simulink model "nms_3Dmodel_mld"  (R2019a)
settings: Solver=ode15s  StartTime=0.0  StopTime=7  FixedStep=1e-3  RelTol=1e-3  AbsTol=1e-4  EnableMultiTasking=on
InitFcn:
  | runScripts;
undefined symbols (not defined in the file or in its folder): ankle_height, c, c_jointstop, CtrlPar_FP, CtrlPar_FP_R, CtrlPar_LL, CtrlPar_St, CtrlPar_St_R, CtrlPar_Sw, CtrlPar_Sw_R, CtrlPar_theta0, CtrlPar_Tr, CtrlPar_Tr_R, D12_F, D12_S, D12_T, D12z_T, D13_F, D1G_F, D1G_HAT, D1G_S, D1G_T, D1Gy_F, d_fBall, d_fHeel, DeltaThRef, dt, eref, FmaxBFSH, FmaxGAS, FmaxGLU, FmaxHAB, FmaxHAD, FmaxHAM, FmaxHFL, FmaxRF, FmaxSOL, FmaxTA, FmaxVAS, In_F, In_HAT, In_S, In_T, init_a_tgt, init_a_tgtR, Inx_F, Inx_HAT, Inx_S, Inx_T, Iny_F, Iny_HAT, Iny_S, Iny_T, K, k_gn, k_gt, k_pressure, leg_l, LongDelay, LongLoopDelay ... (+139)
libraries: mblibv1 x89, simulink x44, simulink_extras x38
(part 2 of 13)

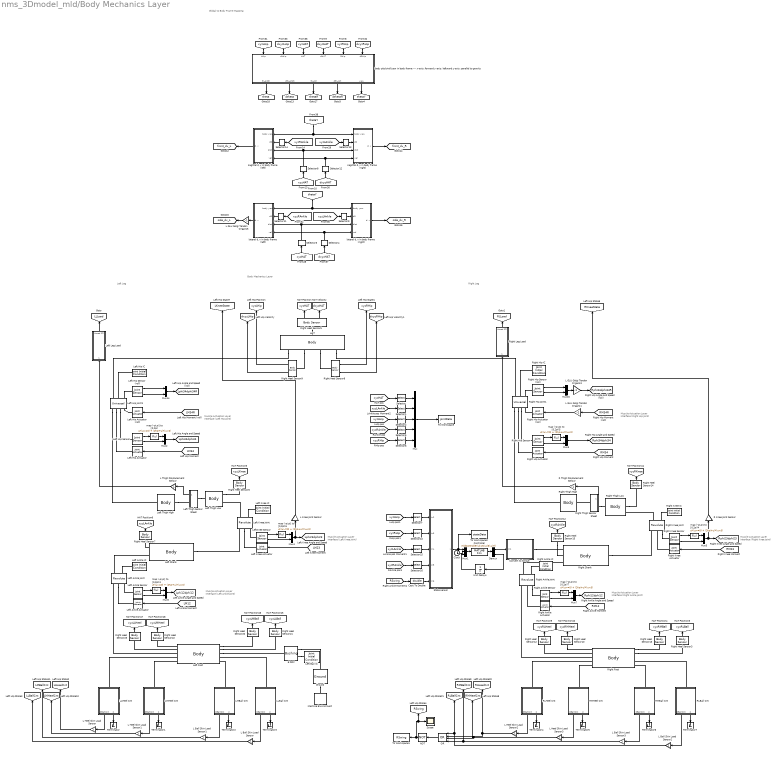
== system nms_3Dmodel_mld/Body Mechanics Layer ==
  note: Body Mechanics Layer
  note: Left Leg
  note: Right Leg
  note: Muscle Actuation
      | Layer Interface
      | (Left Hip Joint)
  note: Muscle Actuation
      | Layer Interface
      | (Left Knee Joint)
  note: Muscle Actuation
      | Layer Interface
      | (Left Ankle Joint)
  note: Muscle Actuation
      | Layer Interface
      | (Right Ankle Joint)
  note: Muscle Actuation
      | Layer Interface
      | (Right Knee Joint)
  note: Muscle Actuation
      | Layer Interface
      | (Right Hip Joint)
  note: Global to Body Frame Mapping
  6 DOF : mblibv1/Joints/Bushing  LConnTagsString=__newl0|SA1  RConnTagsString=__newr0  UpdateFromCAD=off  NumSAPorts=1  CutJoint=off  MarkAsCut=off  Primitives=prismatic_prismatic_prismatic  PrimitiveProps=P1$World$[1 0 0]$prismatic#P2$World$[0 1 0]$prismatic#P3$World$[0 0 1]$prismatic#R1$World$[1 0 0]$revolute#R2$World$[0 1 0]$revolute#R3$World$[0 0 1]$revolute  DialogClass=JointBlock  P1Axis=[1 0 0]  P2Axis=[0 1 0]  P3Axis=[0 0 1]  R1Axis=[1 0 0]  R2Axis=[0 1 0]  R3Axis=[0 0 1]
      settings: SourceProductName=Simscape Multibody  SourceProductBaseCode=MS
  Cast To Double : DataTypeConversion  OutDataTypeStr=double
  Clock : Clock
  Controller : MATLABFcn  MATLABFcn=mldController(u(1:5),u(6),u(7))  OutputDimensions=2  SampleTime=0.01
  "Convert to torque " : Subsystem
  Demux : Demux  Outputs=2
  Ground : mblibv1/Bodies/Ground  UpdateFromCAD=off  LeftPortType=env  RightPortType=workingframe  PhysicalDomain=Mechanical  DialogClass=GroundBlock  CoordPosition=[0 0 0]  CoordPositionUnits=m  StateVectorMgrId=1  MachineId=[2 0]  ShowEnvPort=on  ParameterChecksum=[2753857904, 2875425358, 3568229323, 1209649953]  TopologyChecksum=[3539625464, 3223322067, 2116753285, 3317004890]
      settings: SourceProductName=Simscape Multibody  SourceProductBaseCode=MS
  HAT : mblibv1/Bodies/Body  LConnTagsString=CG  RConnTagsString=CS1|CS2|CS3|CS4  UpdateFromCAD=off  DialogClass=MechanicalBodyBlock  Mass=m_HAT  MassUnits=kg  InertiaUnits=kg*m^2  Inertia=[Inx_HAT 0 0; 0 Iny_HAT 0; 0 0 In_HAT]  Shape=Cylinder  ShapeDims=[1 1]  ShapeUnits=m  ShapeUse=false  Density=1  DensityUnits=kg/m^3  DensityUse=false  GraphicsMode=MACHINE_DEFAULT  BodyColorSelMode=MACHINE_DEFAULT  BodyColor=[1 0 0]  AttachedToCS=CG  CG=Left$CG$[D1G_HAT 0 D12z_T]$CS1$CS1$m$[0 0 0]$Euler X-Y-Z$deg$WORLD$true$none  WorkingFrames=Left$CS5$[0.8 0 D12z_T]$CS1$CS1$m$[0 0 0]$Euler X-Y-Z$deg$WORLD$false$none#Right$CS1$[0 0 0]$ADJOINING$ADJOINING$m$[0 0 0]$Euler X-Y-Z$deg$WORLD$true$none#Right$CS2$[0 0 0]$CS1$CS1$m$[0 0 0]$Euler X-Y-Z$deg$WORLD$true$none#Right$CS3$[0 0 0]$CS4$CS4$m$[0 0 0]$Euler X-Y-Z$deg$WORLD$true$none#Right$CS4$[0 0 2*D12z_T]$CS1$CS1$m$[0 0 0]$Euler X-Y-Z$deg$WORLD$true$none  CGPos=[D1G_HAT 0 D12z_T]  CGRot=[0 0 0]  CS0Pos=[]  CS0Rot=[]  CS1Pos=[0 0 0]  CS1Rot=[0 0 0]  CS2Pos=[0 0 0]  CS2Rot=[0 0 0]  CS3Pos=[0 0 0]  CS3Rot=[0 0 0]  CS4Pos=[0 0 2*D12z_T]  CS4Rot=[0 0 0]  CS5Pos=[0.8 0 D12z_T]  CS5Rot=[0 0 0]  CS6Pos=[]  CS6Rot=[]  CS7Pos=[]  CS7Rot=[]  CS8Pos=[]  CS8Rot=[]  CS9Pos=[]  CS9Rot=[]  CS10Pos=[]  CS10Rot=[]  CS11Pos=[]  CS11Rot=[]  CS12Pos=[]  CS12Rot=[]  CS13Pos=[]  CS13Rot=[]  CS14Pos=[]  CS14Rot=[]  CS15Pos=[]  CS15Rot=[]  CS16Pos=[]  CS16Rot=[]  CS17Pos=[]  CS17Rot=[]  CS18Pos=[]  CS18Rot=[]  CS19Pos=[]  CS19Rot=[]  CS20Pos=[]  CS20Rot=[]
      settings: SourceProductName=Simscape Multibody  SourceProductBaseCode=MS
  L Ball Skin Load Sensor{,1..3} (4 alike) : Gain
  L GLU Golgi Tendon Organs1 : Gain  Gain=-1
  L GLU Golgi Tendon Organs3 : Gain  Gain=-1
  L GLU Golgi Tendon Organs5 : Gain  Gain=-1
  L Heel Skin Load Sensor{,1..3} (4 alike) : Gain
  L Knee Joint Sensor : Gain
  L Thigh Displacement  Sensor : Gain
  LLBall Cnt : Subsystem
  LLHeel Cnt : Subsystem
  LMBall Cnt : Subsystem
  LMHeel Cnt : Subsystem
  Left Ankle Joint : mblibv1/Joints/Revolute  LConnTagsString=__newl0|SA1|SA2  RConnTagsString=__newr0|SA1  UpdateFromCAD=off  NumSAPorts=3  CutJoint=off  MarkAsCut=off  Primitives=revolute  PrimitiveProps=R1$WORLD$[0 0 1]$revolute  DialogClass=JointBlock  R1Axis=[0 0 1]
      settings: SourceProductName=Simscape Multibody  SourceProductBaseCode=MS
  Left Hip Joint1 : mblibv1/Joints/Universal  LConnTagsString=__newl0|SA1|SA2|SA3  RConnTagsString=__newr0|SA1|SA2  UpdateFromCAD=off  NumSAPorts=5  CutJoint=off  MarkAsCut=off  Primitives=prismatic  PrimitiveProps=R1$World$[0 0 1]$revolute#R2$World$[0 1 0]$revolute  DialogClass=JointBlock  R1Axis=[0 0 1]  R2Axis=[0 1 0]
      settings: SourceProductName=Simscape Multibody  SourceProductBaseCode=MS
  Left Knee Joint : mblibv1/Joints/Revolute  LConnTagsString=__newl0|SA1|SA2  RConnTagsString=__newr0|SA1  UpdateFromCAD=off  NumSAPorts=3  CutJoint=off  MarkAsCut=off  Primitives=revolute  PrimitiveProps=R1$WORLD$[0 0 -1]$revolute  DialogClass=JointBlock  R1Axis=[0 0 -1]
      settings: SourceProductName=Simscape Multibody  SourceProductBaseCode=MS
  Left Ankle Actuator : mblibv1/Sensors &  Actuators/Joint Actuator  UpdateFromCAD=off  PhysicalDomain=Mechanical  PortType=blob  ActuationStyle=Force  AngleUnits=deg  ArcVelocityUnits=deg/s  ArcAccelerationUnits=deg/s^2  CoordPositionUnits=m  VelocityUnits=m/s  AccelerationUnits=m/s^2  ForceUnits=N  TorqueUnits=N-m  ActiveIO=on  Width=1  DialogClass=MechanicalActuatorBlock  Primitive=R1  ReferenceFrame=Absolute (INERTIAL)
      settings: SourceProductName=Simscape Multibody  SourceProductBaseCode=MS
  Left Ankle Sensor : mblibv1/Sensors &  Actuators/Joint Sensor  UpdateFromCAD=off  PhysicalDomain=Mechanical  PortType=blob  Muxed=off  Pose=off  Angle=on  AngleUnits=rad  ArcVelocity=on  ArcVelocityUnits=rad/s  ArcAcceleration=off  ArcAccelerationUnits=deg/s^2  CoordPosition=on  CoordPositionUnits=m  Velocity=off  VelocityUnits=m/s  Acceleration=off  AccelerationUnits=m/s^2  Quaternion=on  QuaternionDT=off  QuaternionDDT=off  QuaternionUnits=off  OutputVector=[ 1 1 ]  ActiveIO=on  Width=2  DialogClass=MechanicalSensorBlock  Primitive=R1  Force=off  ForceUnits=N  Torque=off  TorqueUnits=N-m  ReferenceFrame=Absolute (INERTIAL)  ReactionSensedSide=Base  ReactionReferenceFrame=Absolute (World)  ReactionForce=off  ReactionForceUnits=N  ReactionMoment=off  ReactionMomentUnits=N-m
      settings: SourceProductName=Simscape Multibody  SourceProductBaseCode=MS
  Left Ankle IC : mblibv1/Sensors &  Actuators/Joint Initial Condition  UpdateFromCAD=off  LeftPortType=blob  RightPortType=blob  PhysicalDomain=mechanical  DialogClass=InitialConditionBlock  InitialConditions=P1$false$0$m$rad$0$m/s$rad/s#P2$false$0$m$rad$0$m/s$rad/s#P3$false$0$m$rad$0$m/s$rad/s#R1$true$Lphi120$m$rad$0$m/s$rad/s#R2$false$0$m$rad$0$m/s$rad/s#R3$false$0$m$rad$0$m/s$rad/s#S$false$0$m$rad$0$m/s$rad/s  P1PIC=0  P1VIC=0  P2PIC=0  P2VIC=0  P3PIC=0  P3VIC=0  R1PIC=Lphi120  R1VIC=0  R2PIC=0  R2VIC=0  R3PIC=0  R3VIC=0  SPIC=0  SVIC=0
      settings: SourceProductName=Simscape Multibody  SourceProductBaseCode=MS
  Left Ball IC : mblibv1/Sensors &  Actuators/Joint Initial Condition  UpdateFromCAD=off  LeftPortType=blob  RightPortType=blob  PhysicalDomain=mechanical  DialogClass=InitialConditionBlock  InitialConditions=P1$true$x0$m$deg$vx0$m/s$deg/s#P2$true$z0$m$deg$0$m/s$deg/s#P3$true$-y0$m$deg$-vy0$m/s$deg/s#R1$true$roll0$m$rad$0$m/s$rad/s#R2$true$yaw0$m$rad$0$m/s$rad/s#R3$false$0$m$rad$0$m/s$rad/s#S$false$0$m$deg$0$m/s$deg/s  P1PIC=x0  P1VIC=vx0  P2PIC=z0  P2VIC=0  P3PIC=-y0  P3VIC=-vy0  R1PIC=roll0  R1VIC=0  R2PIC=yaw0  R2VIC=0  R3PIC=0  R3VIC=0  SPIC=0  SVIC=0
      settings: SourceProductName=Simscape Multibody  SourceProductBaseCode=MS
  Left Foot : mblibv1/Bodies/Body  LConnTagsString=CS3|CS4|CS1|CS5|CS6  RConnTagsString=CS7|CS8|CS2|CS9|CS10  UpdateFromCAD=off  DialogClass=MechanicalBodyBlock  Mass=m_F  MassUnits=kg  InertiaUnits=kg*m^2  Inertia=[Inx_F 0 0; 0 Iny_F 0; 0 0 In_F]  Shape=Cylinder  ShapeDims=[1 1]  ShapeUnits=m  ShapeUse=false  Density=1  DensityUnits=kg/m^3  DensityUse=false  GraphicsMode=MACHINE_DEFAULT  BodyColorSelMode=MACHINE_DEFAULT  BodyColor=[1 0 0]  AttachedToCS=CG  CG=Left$CG$[-D1G_F D1Gy_F 0]$CS1$CS1$m$[0 0 0]$Euler X-Y-Z$deg$WORLD$false$none  WorkingFrames=Left$CS3$[0 0 d_fBall/2]$CS1$CS1$m$[0 0 0]$Euler X-Y-Z$deg$WORLD$true$none#Left$CS4$[0 0 -d_fBall/2]$CS1$CS1$m$[0 0 0]$Euler X-Y-Z$deg$WORLD$true$none#Right$CS7$[-D13_F 0 d_fHeel/2]$CS1$CS1$m$[0 0 0]$Euler X-Y-Z$deg$WORLD$true$none#Right$CS8$[-D13_F 0 -d_fHeel/2]$CS1$CS1$m$[0 0 0]$Euler X-Y-Z$deg$WORLD$true$none#Left$CS1$[0 0 0]$ADJOINING$ADJOINING$m$[0 0 0]$Euler X-Y-Z$deg$WORLD$true$none#Right$CS2$[-D12_F ankle_height 0]$CS1$CS1$m$[0 0 0]$Euler X-Y-Z$deg$WORLD$true$none#Left$CS5$[0 0 0]$CS4$CS4$m$[0 0 0]$Euler X-Y-Z$deg$WORLD$true$none#Left$CS6$[0 0 0]$CS3$CS3$m$[0 0 0]$Euler X-Y-Z$deg$WORLD$true$none#Right$CS9$[0 0 0]$CS8$CS8$m$[0 0 0]$Euler X-Y-Z$deg$WORLD$true$none#Right$CS10$[0 0 0]$CS7$CS7$m$[0 0 0]$Euler X-Y-Z$deg$WORLD$true$none  CGPos=[-D1G_F D1Gy_F 0]  CGRot=[0 0 0]  CS0Pos=[]  CS0Rot=[]  CS1Pos=[0 0 0]  CS1Rot=[0 0 0]  CS2Pos=[-D12_F ankle_height 0]  CS2Rot=[0 0 0]  CS3Pos=[0 0 d_fBall/2]  CS3Rot=[0 0 0]  CS4Pos=[0 0 -d_fBall/2]  CS4Rot=[0 0 0]  CS5Pos=[0 0 0]  CS5Rot=[0 0 0]  CS6Pos=[0 0 0]  CS6Rot=[0 0 0]  CS7Pos=[-D13_F 0 d_fHeel/2]  CS7Rot=[0 0 0]  CS8Pos=[-D13_F 0 -d_fHeel/2]  CS8Rot=[0 0 0]  CS9Pos=[0 0 0]  CS9Rot=[0 0 0]  CS10Pos=[0 0 0]  CS10Rot=[0 0 0]  CS11Pos=[]  CS11Rot=[]  CS12Pos=[]  CS12Rot=[]  CS13Pos=[]  CS13Rot=[]  CS14Pos=[]  CS14Rot=[]  CS15Pos=[]  CS15Rot=[]  CS16Pos=[]  CS16Rot=[]  CS17Pos=[]  CS17Rot=[]  CS18Pos=[]  CS18Rot=[]  CS19Pos=[]  CS19Rot=[]  CS20Pos=[]  CS20Rot=[]
      settings: SourceProductName=Simscape Multibody  SourceProductBaseCode=MS
  Left Hip Actuator : mblibv1/Sensors &  Actuators/Joint Actuator  UpdateFromCAD=off  PhysicalDomain=Mechanical  PortType=blob  ActuationStyle=Force  AngleUnits=deg  ArcVelocityUnits=deg/s  ArcAccelerationUnits=deg/s^2  CoordPositionUnits=m  VelocityUnits=m/s  AccelerationUnits=m/s^2  ForceUnits=N  TorqueUnits=N-m  ActiveIO=on  Width=1  DialogClass=MechanicalActuatorBlock  Primitive=R1  ReferenceFrame=Absolute (INERTIAL)
      settings: SourceProductName=Simscape Multibody  SourceProductBaseCode=MS
  Left Hip Actuator (roll) : mblibv1/Sensors &  Actuators/Joint Actuator  UpdateFromCAD=off  PhysicalDomain=Mechanical  PortType=blob  ActuationStyle=Force  AngleUnits=rad  ArcVelocityUnits=rad/s  ArcAccelerationUnits=rad/s^2  CoordPositionUnits=m  VelocityUnits=m/s  AccelerationUnits=m/s^2  ForceUnits=N  TorqueUnits=N*m  ActiveIO=on  Width=1  DialogClass=MechanicalActuatorBlock  Primitive=R2  ReferenceFrame=Absolute (INERTIAL)
      settings: SourceProductName=Simscape Multibody  SourceProductBaseCode=MS
  Left Hip Sensor : mblibv1/Sensors &  Actuators/Joint Sensor  UpdateFromCAD=off  PhysicalDomain=Mechanical  PortType=blob  Muxed=off  Pose=off  Angle=on  AngleUnits=rad  ArcVelocity=on  ArcVelocityUnits=rad/s  ArcAcceleration=off  ArcAccelerationUnits=deg/s^2  CoordPosition=on  CoordPositionUnits=m  Velocity=on  VelocityUnits=m/s  Acceleration=off  AccelerationUnits=m/s^2  Quaternion=on  QuaternionDT=off  QuaternionDDT=off  QuaternionUnits=off  OutputVector=[ 1 1 ]  ActiveIO=on  Width=2  DialogClass=MechanicalSensorBlock  Primitive=R1  Force=off  ForceUnits=N  Torque=off  TorqueUnits=N-m  ReferenceFrame=Absolute (INERTIAL)  ReactionSensedSide=Base  ReactionReferenceFrame=Absolute (World)  ReactionForce=off  ReactionForceUnits=N  ReactionMoment=off  ReactionMomentUnits=N-m
      settings: SourceProductName=Simscape Multibody  SourceProductBaseCode=MS
  Left Hip Sensor (roll) : mblibv1/Sensors &  Actuators/Joint Sensor  UpdateFromCAD=off  PhysicalDomain=Mechanical  PortType=blob  Muxed=off  Pose=off  Angle=on  AngleUnits=rad  ArcVelocity=on  ArcVelocityUnits=rad/s  ArcAcceleration=off  ArcAccelerationUnits=deg/s^2  CoordPosition=on  CoordPositionUnits=m  Velocity=on  VelocityUnits=m/s  Acceleration=off  AccelerationUnits=m/s^2  Quaternion=on  QuaternionDT=off  QuaternionDDT=off  QuaternionUnits=off  OutputVector=[ 1 1 ]  ActiveIO=on  Width=2  DialogClass=MechanicalSensorBlock  Primitive=R2  Force=off  ForceUnits=N  Torque=off  TorqueUnits=N*m  ReferenceFrame=Absolute (INERTIAL)  ReactionSensedSide=Base  ReactionReferenceFrame=Absolute (World)  ReactionForce=off  ReactionForceUnits=N  ReactionMoment=off  ReactionMomentUnits=N*m
      settings: SourceProductName=Simscape Multibody  SourceProductBaseCode=MS
  Left Hip IC : mblibv1/Sensors &  Actuators/Joint Initial Condition  UpdateFromCAD=off  LeftPortType=blob  RightPortType=blob  PhysicalDomain=mechanical  DialogClass=InitialConditionBlock  InitialConditions=P1$false$0$m$rad$0$m/s$rad/s#P2$false$0$m$rad$0$m/s$rad/s#P3$false$0$m$rad$0$m/s$rad/s#R1$true$Lphi340$m$rad$0$m/s$rad/s#R2$true$Lphi340R$m$rad$0$m/s$rad/s#R3$false$0$m$rad$0$m/s$rad/s#S$false$0$m$rad$0$m/s$rad/s  P1PIC=0  P1VIC=0  P2PIC=0  P2VIC=0  P3PIC=0  P3VIC=0  R1PIC=Lphi340  R1VIC=0  R2PIC=Lphi340R  R2VIC=0  R3PIC=0  R3VIC=0  SPIC=0  SVIC=0
      settings: SourceProductName=Simscape Multibody  SourceProductBaseCode=MS
  Left Knee Actuator : mblibv1/Sensors &  Actuators/Joint Actuator  UpdateFromCAD=off  PhysicalDomain=Mechanical  PortType=blob  ActuationStyle=Force  AngleUnits=deg  ArcVelocityUnits=deg/s  ArcAccelerationUnits=deg/s^2  CoordPositionUnits=m  VelocityUnits=m/s  AccelerationUnits=m/s^2  ForceUnits=N  TorqueUnits=N-m  ActiveIO=on  Width=1  DialogClass=MechanicalActuatorBlock  Primitive=R1  ReferenceFrame=Absolute (INERTIAL)
      settings: SourceProductName=Simscape Multibody  SourceProductBaseCode=MS
  Left Knee IC : mblibv1/Sensors &  Actuators/Joint Initial Condition  UpdateFromCAD=off  LeftPortType=blob  RightPortType=blob  PhysicalDomain=mechanical  DialogClass=InitialConditionBlock  InitialConditions=P1$false$0$m$rad$0$m/s$rad/s#P2$false$0$m$rad$0$m/s$rad/s#P3$false$0$m$rad$0$m/s$rad/s#R1$true$Lphi230$m$rad$0$m/s$deg/s#R2$false$0$m$rad$0$m/s$rad/s#R3$false$0$m$rad$0$m/s$rad/s#S$false$0$m$rad$0$m/s$rad/s  P1PIC=0  P1VIC=0  P2PIC=0  P2VIC=0  P3PIC=0  P3VIC=0  R1PIC=Lphi230  R1VIC=0  R2PIC=0  R2VIC=0  R3PIC=0  R3VIC=0  SPIC=0  SVIC=0
      settings: SourceProductName=Simscape Multibody  SourceProductBaseCode=MS
  Left Leg Load : Subsystem
  Left Shank : mblibv1/Bodies/Body  LConnTagsString=CS3|CS1  RConnTagsString=CS2  UpdateFromCAD=off  DialogClass=MechanicalBodyBlock  Mass=m_S  MassUnits=kg  InertiaUnits=kg*m^2  Inertia=[Inx_S 0 0; 0 Iny_S 0; 0 0 In_S]  Shape=Cylinder  ShapeDims=[1 1]  ShapeUnits=m  ShapeUse=false  Density=1  DensityUnits=kg/m^3  DensityUse=false  GraphicsMode=MACHINE_DEFAULT  BodyColorSelMode=MACHINE_DEFAULT  BodyColor=[1 0 0]  AttachedToCS=CG  CG=Left$CG$[D1G_S 0 0]$CS1$CS1$m$[0 0 0]$Euler X-Y-Z$deg$WORLD$false$none  WorkingFrames=Left$CS3$[0 0 0]$CS1$CS1$m$[0 0 0]$Euler X-Y-Z$deg$WORLD$true$none#Left$CS1$[0 0 0]$ADJOINING$ADJOINING$m$[0 0 0]$Euler X-Y-Z$deg$WORLD$true$none#Right$CS2$[D12_S 0 0]$CS1$CS1$m$[0 0 0]$Euler X-Y-Z$deg$WORLD$true$none  CGPos=[D1G_S 0 0]  CGRot=[0 0 0]  CS0Pos=[]  CS0Rot=[]  CS1Pos=[0 0 0]  CS1Rot=[0 0 0]  CS2Pos=[D12_S 0 0]  CS2Rot=[0 0 0]  CS3Pos=[0 0 0]  CS3Rot=[0 0 0]  CS4Pos=[]  CS4Rot=[]  CS5Pos=[]  CS5Rot=[]  CS6Pos=[]  CS6Rot=[]  CS7Pos=[]  CS7Rot=[]  CS8Pos=[]  CS8Rot=[]  CS9Pos=[]  CS9Rot=[]  CS10Pos=[]  CS10Rot=[]  CS11Pos=[]  CS11Rot=[]  CS12Pos=[]  CS12Rot=[]  CS13Pos=[]  CS13Rot=[]  CS14Pos=[]  CS14Rot=[]  CS15Pos=[]  CS15Rot=[]  CS16Pos=[]  CS16Rot=[]  CS17Pos=[]  CS17Rot=[]  CS18Pos=[]  CS18Rot=[]  CS19Pos=[]  CS19Rot=[]  CS20Pos=[]  CS20Rot=[]
      settings: SourceProductName=Simscape Multibody  SourceProductBaseCode=MS
  Left Thigh Sensor Sheet : Subsystem
  Left Thigh High : mblibv1/Bodies/Body  LConnTagsString=CS2  RConnTagsString=CS1  UpdateFromCAD=off  DialogClass=MechanicalBodyBlock  Mass=m_T*(1-ThPos)  MassUnits=kg  InertiaUnits=kg*m^2  Inertia=[Inx_T*(1-ThPos) 0 0; 0 Iny_T*(1-ThPos)^3 0; 0 0 In_T*(1-ThPos)^3]  Shape=Cylinder  ShapeDims=[1 1]  ShapeUnits=m  ShapeUse=false  Density=1  DensityUnits=kg/m^3  DensityUse=false  GraphicsMode=MACHINE_DEFAULT  BodyColorSelMode=MACHINE_DEFAULT  BodyColor=[1 0 0]  AttachedToCS=CG  CG=Left$CG$[-D1G_T*(1-ThPos) 0 0]$CS1$CS1$m$[0 0 0]$Euler X-Y-Z$deg$WORLD$false$none  WorkingFrames=Right$CS1$[0 0 0]$ADJOINING$ADJOINING$m$[0 0 0]$Euler X-Y-Z$deg$WORLD$true$none#Left$CS2$[-D12_T*(1-ThPos) 0 0]$CS1$CS1$m$[0 0 0]$Euler X-Y-Z$deg$WORLD$true$none  CGPos=[-D1G_T*(1-ThPos) 0 0]  CGRot=[0 0 0]  CS0Pos=[]  CS0Rot=[]  CS1Pos=[0 0 0]  CS1Rot=[0 0 0]  CS2Pos=[-D12_T*(1-ThPos) 0 0]  CS2Rot=[0 0 0]  CS3Pos=[]  CS3Rot=[]  CS4Pos=[]  CS4Rot=[]  CS5Pos=[]  CS5Rot=[]  CS6Pos=[]  CS6Rot=[]  CS7Pos=[]  CS7Rot=[]  CS8Pos=[]  CS8Rot=[]  CS9Pos=[]  CS9Rot=[]  CS10Pos=[]  CS10Rot=[]  CS11Pos=[]  CS11Rot=[]  CS12Pos=[]  CS12Rot=[]  CS13Pos=[]  CS13Rot=[]  CS14Pos=[]  CS14Rot=[]  CS15Pos=[]  CS15Rot=[]  CS16Pos=[]  CS16Rot=[]  CS17Pos=[]  CS17Rot=[]  CS18Pos=[]  CS18Rot=[]  CS19Pos=[]  CS19Rot=[]  CS20Pos=[]  CS20Rot=[]
      settings: SourceProductName=Simscape Multibody  SourceProductBaseCode=MS
  Left Thigh Low : mblibv1/Bodies/Body  LConnTagsString=CS2  RConnTagsString=CS3|CS1  UpdateFromCAD=off  DialogClass=MechanicalBodyBlock  Mass=m_T*ThPos  MassUnits=kg  InertiaUnits=kg*m^2  Inertia=[Inx_T*ThPos 0 0; 0 Iny_T*(ThPos)^3 0; 0 0 In_T*(ThPos)^3]  Shape=Cylinder  ShapeDims=[1 1]  ShapeUnits=m  ShapeUse=false  Density=1  DensityUnits=kg/m^3  DensityUse=false  GraphicsMode=MACHINE_DEFAULT  BodyColorSelMode=MACHINE_DEFAULT  BodyColor=[1 0 0]  AttachedToCS=CG  CG=Left$CG$[-D1G_T*ThPos 0 0]$CS1$CS1$m$[0 0 0]$Euler X-Y-Z$deg$WORLD$false$none  WorkingFrames=Right$CS3$[0 0 0]$CS1$CS1$m$[0 0 0]$Euler X-Y-Z$deg$WORLD$true$none#Right$CS1$[0 0 0]$ADJOINING$ADJOINING$m$[0 0 0]$Euler X-Y-Z$deg$WORLD$true$none#Left$CS2$[-D12_T*ThPos 0 0]$CS1$CS1$m$[0 0 0]$Euler X-Y-Z$deg$WORLD$true$none  CGPos=[-D1G_T*ThPos 0 0]  CGRot=[0 0 0]  CS0Pos=[]  CS0Rot=[]  CS1Pos=[0 0 0]  CS1Rot=[0 0 0]  CS2Pos=[-D12_T*ThPos 0 0]  CS2Rot=[0 0 0]  CS3Pos=[0 0 0]  CS3Rot=[0 0 0]  CS4Pos=[]  CS4Rot=[]  CS5Pos=[]  CS5Rot=[]  CS6Pos=[]  CS6Rot=[]  CS7Pos=[]  CS7Rot=[]  CS8Pos=[]  CS8Rot=[]  CS9Pos=[]  CS9Rot=[]  CS10Pos=[]  CS10Rot=[]  CS11Pos=[]  CS11Rot=[]  CS12Pos=[]  CS12Rot=[]  CS13Pos=[]  CS13Rot=[]  CS14Pos=[]  CS14Rot=[]  CS15Pos=[]  CS15Rot=[]  CS16Pos=[]  CS16Rot=[]  CS17Pos=[]  CS17Rot=[]  CS18Pos=[]  CS18Rot=[]  CS19Pos=[]  CS19Rot=[]  CS20Pos=[]  CS20Rot=[]
      settings: SourceProductName=Simscape Multibody  SourceProductBaseCode=MS
  LeftKnee Sensor : mblibv1/Sensors &  Actuators/Joint Sensor  UpdateFromCAD=off  PhysicalDomain=Mechanical  PortType=blob  Muxed=off  Pose=off  Angle=on  AngleUnits=rad  ArcVelocity=on  ArcVelocityUnits=rad/s  ArcAcceleration=off  ArcAccelerationUnits=deg/s^2  CoordPosition=on  CoordPositionUnits=m  Velocity=off  VelocityUnits=m/s  Acceleration=off  AccelerationUnits=m/s^2  Quaternion=on  QuaternionDT=off  QuaternionDDT=off  QuaternionUnits=off  OutputVector=[ 1 1 ]  ActiveIO=on  Width=2  DialogClass=MechanicalSensorBlock  Primitive=R1  Force=off  ForceUnits=N  Torque=off  TorqueUnits=N-m  ReferenceFrame=Absolute (INERTIAL)  ReactionSensedSide=Base  ReactionReferenceFrame=Absolute (World)  ReactionForce=off  ReactionForceUnits=N  ReactionMoment=off  ReactionMomentUnits=N-m
      settings: SourceProductName=Simscape Multibody  SourceProductBaseCode=MS
  Machine Environment : mblibv1/Bodies/Machine Environment  Tag=Factory ground  PortType=env  PhysicalDomain=Mechanical  DialogTemplateClass=MECH.MachineEnvironment  SyncWhenCopied=off  Gravity=[0 -9.81 0]  GravityUnits=m/s^2  GravityAsSignal=off  Dimensionality=3D Only  AnalysisType=Forward dynamics  LinearAssemblyTolerance=1e-3  LinearAssemblyToleranceUnits=m  AngularAssemblyTolerance=1e-3  AngularAssemblyToleranceUnits=rad  ConstraintSolverType=Tolerancing  ConstraintRelTolerance=1e-3  ConstraintAbsTolerance=1e-3  UseRobustSingularityHandling=off  RedundancyAnalysisToleranceType=Automatically select tolerance  RedundancyAnalysisTolerance=1e-14  StatePerturbationType=Fixed  PerturbationSize=1e-3  VisualizeMachine=on  BodyVisualizationType=Use model default body geometries  BodyColorSelMode=Use model default  DefaultBodyColor=[1 0 0]
      settings: SourceProductName=Simscape Multibody  SourceProductBaseCode=MS
  Mux : Mux  Inputs=5
  Mux1 : Mux  Inputs=3
  Mux{2..7,14..15} (8 alike) : Mux  Inputs=2
  NOT : Logic  Operator=NOT  IconShape=distinctive  AllPortsSameDT=off  OutDataTypeStr=boolean
  OR : Logic  Operator=OR  Inputs=4  IconShape=distinctive  AllPortsSameDT=off  OutDataTypeStr=boolean
  R Knee Joint Sensor : Gain
  R Thigh Displacement  Sensor : Gain  Gain=-1
  RLBall Cnt : Subsystem
  RLHeel Cnt : Subsystem
  RMBall Cnt : Subsystem
  RMHeel Cnt : Subsystem
  Right Ankle Joint : mblibv1/Joints/Revolute  LConnTagsString=__newl0|SA1|SA2  RConnTagsString=__newr0|SA1  UpdateFromCAD=off  NumSAPorts=3  CutJoint=off  MarkAsCut=off  Primitives=revolute  PrimitiveProps=R1$WORLD$[0 0 1]$revolute  DialogClass=JointBlock  R1Axis=[0 0 1]
      settings: SourceProductName=Simscape Multibody  SourceProductBaseCode=MS
  Right Hip Joint1 : mblibv1/Joints/Universal  LConnTagsString=__newl0|SA1|SA2|SA3  RConnTagsString=__newr0|SA1|SA2  UpdateFromCAD=off  NumSAPorts=5  CutJoint=off  MarkAsCut=off  Primitives=prismatic  PrimitiveProps=R1$World$[0 0 1]$revolute#R2$World$[0 1 0]$revolute  DialogClass=JointBlock  R1Axis=[0 0 1]  R2Axis=[0 1 0]
      settings: SourceProductName=Simscape Multibody  SourceProductBaseCode=MS
  Right Knee Joint : mblibv1/Joints/Revolute  LConnTagsString=__newl0|SA1|SA2  RConnTagsString=__newr0|SA1  UpdateFromCAD=off  NumSAPorts=3  CutJoint=off  MarkAsCut=off  Primitives=revolute  PrimitiveProps=R1$WORLD$[0 0 -1]$revolute  DialogClass=JointBlock  R1Axis=[0 0 -1]
      settings: SourceProductName=Simscape Multibody  SourceProductBaseCode=MS
  Right Ankle Actuator : mblibv1/Sensors &  Actuators/Joint Actuator  UpdateFromCAD=off  PhysicalDomain=Mechanical  PortType=blob  ActuationStyle=Force  AngleUnits=deg  ArcVelocityUnits=deg/s  ArcAccelerationUnits=deg/s^2  CoordPositionUnits=m  VelocityUnits=m/s  AccelerationUnits=m/s^2  ForceUnits=N  TorqueUnits=N-m  ActiveIO=on  Width=1  DialogClass=MechanicalActuatorBlock  Primitive=R1  ReferenceFrame=Absolute (INERTIAL)
      settings: SourceProductName=Simscape Multibody  SourceProductBaseCode=MS
  Right Ankle Sensor : mblibv1/Sensors &  Actuators/Joint Sensor  UpdateFromCAD=off  PhysicalDomain=Mechanical  PortType=blob  Muxed=off  Pose=off  Angle=on  AngleUnits=rad  ArcVelocity=on  ArcVelocityUnits=rad/s  ArcAcceleration=off  ArcAccelerationUnits=deg/s^2  CoordPosition=on  CoordPositionUnits=m  Velocity=off  VelocityUnits=m/s  Acceleration=off  AccelerationUnits=m/s^2  Quaternion=on  QuaternionDT=off  QuaternionDDT=off  QuaternionUnits=off  OutputVector=[ 1 1 ]  ActiveIO=on  Width=2  DialogClass=MechanicalSensorBlock  Primitive=R1  Force=off  ForceUnits=N  Torque=off  TorqueUnits=N-m  ReferenceFrame=Absolute (INERTIAL)  ReactionSensedSide=Base  ReactionReferenceFrame=Absolute (World)  ReactionForce=off  ReactionForceUnits=N  ReactionMoment=off  ReactionMomentUnits=N-m
      settings: SourceProductName=Simscape Multibody  SourceProductBaseCode=MS
  Right Ankle IC : mblibv1/Sensors &  Actuators/Joint Initial Condition  UpdateFromCAD=off  LeftPortType=blob  RightPortType=blob  PhysicalDomain=mechanical  DialogClass=InitialConditionBlock  InitialConditions=P1$false$0$m$rad$0$m/s$rad/s#P2$false$0$m$rad$0$m/s$rad/s#P3$false$0$m$rad$0$m/s$rad/s#R1$true$Rphi120$m$rad$0$m/s$rad/s#R2$false$0$m$rad$0$m/s$rad/s#R3$false$0$m$rad$0$m/s$rad/s#S$false$0$m$rad$0$m/s$rad/s  P1PIC=0  P1VIC=0  P2PIC=0  P2VIC=0  P3PIC=0  P3VIC=0  R1PIC=Rphi120  R1VIC=0  R2PIC=0  R2VIC=0  R3PIC=0  R3VIC=0  SPIC=0  SVIC=0
      settings: SourceProductName=Simscape Multibody  SourceProductBaseCode=MS
  Right Foot : mblibv1/Bodies/Body  LConnTagsString=CS3|CS4|CS2|CS5|CS6  RConnTagsString=CS7|CS8|CS1|CS9|CS10  UpdateFromCAD=off  DialogClass=MechanicalBodyBlock  Mass=m_F  MassUnits=kg  InertiaUnits=kg*m^2  Inertia=[Inx_F 0 0; 0 Iny_F 0; 0 0 In_F]  Shape=Cylinder  ShapeDims=[1 1]  ShapeUnits=m  ShapeUse=false  Density=1  DensityUnits=kg/m^3  DensityUse=false  GraphicsMode=MACHINE_DEFAULT  BodyColorSelMode=MACHINE_DEFAULT  BodyColor=[1 0 0]  AttachedToCS=CG  CG=Left$CG$[-D1G_F D1Gy_F 0]$CS2$CS2$m$[0 0 0]$Euler X-Y-Z$deg$WORLD$false$none  WorkingFrames=Left$CS3$[0 0 -d_fBall/2]$CS2$CS2$m$[0 0 0]$Euler X-Y-Z$deg$WORLD$true$none#Left$CS4$[0 0 d_fBall/2]$CS2$CS2$m$[0 0 0]$Euler X-Y-Z$deg$WORLD$true$none#Right$CS7$[-D13_F 0 -d_fHeel/2]$CS2$CS2$m$[0 0 0]$Euler X-Y-Z$deg$WORLD$true$none#Right$CS8$[-D13_F 0 d_fHeel/2]$CS2$CS2$m$[0 0 0]$Euler X-Y-Z$deg$WORLD$true$none#Right$CS1$[0 0 0]$ADJOINING$ADJOINING$m$[0 0 0]$Euler X-Y-Z$deg$WORLD$true$none#Left$CS2$[D12_F -ankle_height 0]$CS1$CS1$m$[0 0 0]$Euler X-Y-Z$deg$WORLD$true$none#Left$CS5$[0 0 0]$CS4$CS4$m$[0 0 0]$Euler X-Y-Z$deg$WORLD$true$none#Left$CS6$[0 0 0]$CS3$CS3$m$[0 0 0]$Euler X-Y-Z$deg$WORLD$true$none#Right$CS9$[0 0 0]$CS8$CS8$m$[0 0 0]$Euler X-Y-Z$deg$WORLD$true$none#Right$CS10$[0 0 0]$CS7$CS7$m$[0 0 0]$Euler X-Y-Z$deg$WORLD$true$none  CGPos=[-D1G_F D1Gy_F 0]  CGRot=[0 0 0]  CS0Pos=[]  CS0Rot=[]  CS1Pos=[0 0 0]  CS1Rot=[0 0 0]  CS2Pos=[D12_F -ankle_height 0]  CS2Rot=[0 0 0]  CS3Pos=[0 0 -d_fBall/2]  CS3Rot=[0 0 0]  CS4Pos=[0 0 d_fBall/2]  CS4Rot=[0 0 0]  CS5Pos=[0 0 0]  CS5Rot=[0 0 0]  CS6Pos=[0 0 0]  CS6Rot=[0 0 0]  CS7Pos=[-D13_F 0 -d_fHeel/2]  CS7Rot=[0 0 0]  CS8Pos=[-D13_F 0 d_fHeel/2]  CS8Rot=[0 0 0]  CS9Pos=[0 0 0]  CS9Rot=[0 0 0]  CS10Pos=[0 0 0]  CS10Rot=[0 0 0]  CS11Pos=[]  CS11Rot=[]  CS12Pos=[]  CS12Rot=[]  CS13Pos=[]  CS13Rot=[]  CS14Pos=[]  CS14Rot=[]  CS15Pos=[]  CS15Rot=[]  CS16Pos=[]  CS16Rot=[]  CS17Pos=[]  CS17Rot=[]  CS18Pos=[]  CS18Rot=[]  CS19Pos=[]  CS19Rot=[]  CS20Pos=[]  CS20Rot=[]
      settings: SourceProductName=Simscape Multibody  SourceProductBaseCode=MS
  Right Heel Sensor{3,6..7,10,12..15,20..23} (12 alike) : mblibv1/Sensors &  Actuators/Body Sensor  UpdateFromCAD=off  PhysicalDomain=Mechanical  PortType=blob  Muxed=off  Pose=off  Angle=on  AngleUnits=deg  ArcVelocity=off  ArcVelocityUnits=deg/s  ArcAcceleration=off  ArcAccelerationUnits=deg/s^2  CoordPosition=on  CoordPositionUnits=m  Velocity=off  VelocityUnits=m/s  Acceleration=off  AccelerationUnits=m/s^2  Quaternion=on  QuaternionDT=off  QuaternionDDT=off  QuaternionUnits=off  OutputVector=[ 3 3 ]  ActiveIO=on  Width=3  DialogClass=MechanicalSensorBlock  ReferenceFrame=Absolute (World)
      settings: SourceProductName=Simscape Multibody  SourceProductBaseCode=MS
  Right Heel Sensor5 : mblibv1/Sensors &  Actuators/Body Sensor  UpdateFromCAD=off  PhysicalDomain=Mechanical  PortType=blob  Muxed=off  Pose=off  Angle=on  AngleUnits=deg  ArcVelocity=off  ArcVelocityUnits=deg/s  ArcAcceleration=off  ArcAccelerationUnits=deg/s^2  CoordPosition=on  CoordPositionUnits=m  Velocity=on  VelocityUnits=m/s  Acceleration=off  AccelerationUnits=m/s^2  Quaternion=on  QuaternionDT=off  QuaternionDDT=off  QuaternionUnits=off  OutputVector=[ 3 3 ]  ActiveIO=on  Width=6  DialogClass=MechanicalSensorBlock  ReferenceFrame=Absolute (World)
      settings: SourceProductName=Simscape Multibody  SourceProductBaseCode=MS
  Right Heel Sensor8 : mblibv1/Sensors &  Actuators/Body Sensor  UpdateFromCAD=off  PhysicalDomain=Mechanical  PortType=blob  Muxed=off  Pose=off  Angle=on  AngleUnits=deg  ArcVelocity=off  ArcVelocityUnits=deg/s  ArcAcceleration=off  ArcAccelerationUnits=deg/s^2  CoordPosition=on  CoordPositionUnits=m  Velocity=on  VelocityUnits=m/s  Acceleration=off  AccelerationUnits=m/s^2  Quaternion=on  QuaternionDT=off  QuaternionDDT=off  QuaternionUnits=off  OutputVector=[ 3 3 ]  ActiveIO=on  Width=6  DialogClass=MechanicalSensorBlock  ReferenceFrame=Absolute (World)
      settings: SourceProductName=Simscape Multibody  SourceProductBaseCode=MS
  Right Heel Sensor9 : mblibv1/Sensors &  Actuators/Body Sensor  UpdateFromCAD=off  PhysicalDomain=Mechanical  PortType=blob  Muxed=off  Pose=off  Angle=on  AngleUnits=deg  ArcVelocity=off  ArcVelocityUnits=deg/s  ArcAcceleration=off  ArcAccelerationUnits=deg/s^2  CoordPosition=on  CoordPositionUnits=m  Velocity=on  VelocityUnits=m/s  Acceleration=off  AccelerationUnits=m/s^2  Quaternion=on  QuaternionDT=off  QuaternionDDT=off  QuaternionUnits=off  OutputVector=[ 3 3 ]  ActiveIO=on  Width=6  DialogClass=MechanicalSensorBlock  ReferenceFrame=Absolute (World)
      settings: SourceProductName=Simscape Multibody  SourceProductBaseCode=MS
  Right Hip Actuator : mblibv1/Sensors &  Actuators/Joint Actuator  UpdateFromCAD=off  PhysicalDomain=Mechanical  PortType=blob  ActuationStyle=Force  AngleUnits=deg  ArcVelocityUnits=deg/s  ArcAccelerationUnits=deg/s^2  CoordPositionUnits=m  VelocityUnits=m/s  AccelerationUnits=m/s^2  ForceUnits=N  TorqueUnits=N-m  ActiveIO=on  Width=1  DialogClass=MechanicalActuatorBlock  Primitive=R1  ReferenceFrame=Absolute (INERTIAL)
      settings: SourceProductName=Simscape Multibody  SourceProductBaseCode=MS
  Right Hip Actuator (roll) : mblibv1/Sensors &  Actuators/Joint Actuator  UpdateFromCAD=off  PhysicalDomain=Mechanical  PortType=blob  ActuationStyle=Force  AngleUnits=rad  ArcVelocityUnits=rad/s  ArcAccelerationUnits=rad/s^2  CoordPositionUnits=m  VelocityUnits=m/s  AccelerationUnits=m/s^2  ForceUnits=N  TorqueUnits=N*m  ActiveIO=on  Width=1  DialogClass=MechanicalActuatorBlock  Primitive=R2  ReferenceFrame=Absolute (INERTIAL)
      settings: SourceProductName=Simscape Multibody  SourceProductBaseCode=MS
  Right Hip Sensor : mblibv1/Sensors &  Actuators/Joint Sensor  UpdateFromCAD=off  PhysicalDomain=Mechanical  PortType=blob  Muxed=off  Pose=off  Angle=on  AngleUnits=rad  ArcVelocity=on  ArcVelocityUnits=rad/s  ArcAcceleration=off  ArcAccelerationUnits=deg/s^2  CoordPosition=on  CoordPositionUnits=m  Velocity=on  VelocityUnits=m/s  Acceleration=off  AccelerationUnits=m/s^2  Quaternion=on  QuaternionDT=off  QuaternionDDT=off  QuaternionUnits=off  OutputVector=[ 1 1 ]  ActiveIO=on  Width=2  DialogClass=MechanicalSensorBlock  Primitive=R1  Force=off  ForceUnits=N  Torque=off  TorqueUnits=N-m  ReferenceFrame=Absolute (INERTIAL)  ReactionSensedSide=Base  ReactionReferenceFrame=Absolute (World)  ReactionForce=off  ReactionForceUnits=N  ReactionMoment=off  ReactionMomentUnits=N-m
      settings: SourceProductName=Simscape Multibody  SourceProductBaseCode=MS
  Right Hip Sensor (roll) : mblibv1/Sensors &  Actuators/Joint Sensor  UpdateFromCAD=off  PhysicalDomain=Mechanical  PortType=blob  Muxed=off  Pose=off  Angle=on  AngleUnits=rad  ArcVelocity=on  ArcVelocityUnits=rad/s  ArcAcceleration=off  ArcAccelerationUnits=deg/s^2  CoordPosition=on  CoordPositionUnits=m  Velocity=on  VelocityUnits=m/s  Acceleration=off  AccelerationUnits=m/s^2  Quaternion=on  QuaternionDT=off  QuaternionDDT=off  QuaternionUnits=off  OutputVector=[ 1 1 ]  ActiveIO=on  Width=2  DialogClass=MechanicalSensorBlock  Primitive=R2  Force=off  ForceUnits=N  Torque=off  TorqueUnits=N*m  ReferenceFrame=Absolute (INERTIAL)  ReactionSensedSide=Base  ReactionReferenceFrame=Absolute (World)  ReactionForce=off  ReactionForceUnits=N  ReactionMoment=off  ReactionMomentUnits=N*m
      settings: SourceProductName=Simscape Multibody  SourceProductBaseCode=MS
  Right Hip IC : mblibv1/Sensors &  Actuators/Joint Initial Condition  UpdateFromCAD=off  LeftPortType=blob  RightPortType=blob  PhysicalDomain=mechanical  DialogClass=InitialConditionBlock  InitialConditions=P1$false$0$m$rad$0$m/s$rad/s#P2$false$0$m$rad$0$m/s$rad/s#P3$false$0$m$rad$0$m/s$rad/s#R1$true$Rphi340$m$rad$0$m/s$rad/s#R2$true$-Rphi340R$m$rad$0$m/s$rad/s#R3$false$0$m$rad$0$m/s$rad/s#S$false$0$m$rad$0$m/s$rad/s  P1PIC=0  P1VIC=0  P2PIC=0  P2VIC=0  P3PIC=0  P3VIC=0  R1PIC=Rphi340  R1VIC=0  R2PIC=-Rphi340R  R2VIC=0  R3PIC=0  R3VIC=0  SPIC=0  SVIC=0
      settings: SourceProductName=Simscape Multibody  SourceProductBaseCode=MS
  Right Knee Actuator : mblibv1/Sensors &  Actuators/Joint Actuator  UpdateFromCAD=off  PhysicalDomain=Mechanical  PortType=blob  ActuationStyle=Force  AngleUnits=deg  ArcVelocityUnits=deg/s  ArcAccelerationUnits=deg/s^2  CoordPositionUnits=m  VelocityUnits=m/s  AccelerationUnits=m/s^2  ForceUnits=N  TorqueUnits=N-m  ActiveIO=on  Width=1  DialogClass=MechanicalActuatorBlock  Primitive=R1  ReferenceFrame=Absolute (INERTIAL)
      settings: SourceProductName=Simscape Multibody  SourceProductBaseCode=MS
  Right Knee Sensor : mblibv1/Sensors &  Actuators/Joint Sensor  UpdateFromCAD=off  PhysicalDomain=Mechanical  PortType=blob  Muxed=off  Pose=off  Angle=on  AngleUnits=rad  ArcVelocity=on  ArcVelocityUnits=rad/s  ArcAcceleration=off  ArcAccelerationUnits=deg/s^2  CoordPosition=on  CoordPositionUnits=m  Velocity=off  VelocityUnits=m/s  Acceleration=off  AccelerationUnits=m/s^2  Quaternion=on  QuaternionDT=off  QuaternionDDT=off  QuaternionUnits=off  OutputVector=[ 1 1 ]  ActiveIO=on  Width=2  DialogClass=MechanicalSensorBlock  Primitive=R1  Force=off  ForceUnits=N  Torque=off  TorqueUnits=N-m  ReferenceFrame=Absolute (INERTIAL)  ReactionSensedSide=Base  ReactionReferenceFrame=Absolute (World)  ReactionForce=off  ReactionForceUnits=N  ReactionMoment=off  ReactionMomentUnits=N-m
      settings: SourceProductName=Simscape Multibody  SourceProductBaseCode=MS
  Right Knee IC : mblibv1/Sensors &  Actuators/Joint Initial Condition  UpdateFromCAD=off  LeftPortType=blob  RightPortType=blob  PhysicalDomain=mechanical  DialogClass=InitialConditionBlock  InitialConditions=P1$false$0$m$rad$0$m/s$rad/s#P2$false$0$m$rad$0$m/s$rad/s#P3$false$0$m$rad$0$m/s$rad/s#R1$true$Rphi230$m$rad$0$m/s$rad/s#R2$false$0$m$rad$0$m/s$rad/s#R3$false$0$m$rad$0$m/s$rad/s#S$false$0$m$rad$0$m/s$rad/s  P1PIC=0  P1VIC=0  P2PIC=0  P2VIC=0  P3PIC=0  P3VIC=0  R1PIC=Rphi230  R1VIC=0  R2PIC=0  R2VIC=0  R3PIC=0  R3VIC=0  SPIC=0  SVIC=0
      settings: SourceProductName=Simscape Multibody  SourceProductBaseCode=MS
  Right Leg Load : Subsystem
  Right Shank : mblibv1/Bodies/Body  LConnTagsString=CG|CS3|CS2  RConnTagsString=CS1  UpdateFromCAD=off  DialogClass=MechanicalBodyBlock  Mass=m_S  MassUnits=kg  InertiaUnits=kg*m^2  Inertia=[Inx_S 0 0; 0 Iny_S 0; 0 0 In_S]  Shape=Cylinder  ShapeDims=[1 1]  ShapeUnits=m  ShapeUse=false  Density=1  DensityUnits=kg/m^3  DensityUse=false  GraphicsMode=MACHINE_DEFAULT  BodyColorSelMode=MACHINE_DEFAULT  BodyColor=[1 0 0]  AttachedToCS=CG  CG=Left$CG$[D1G_S 0 0]$CS2$CS2$m$[0 0 0]$Euler X-Y-Z$deg$WORLD$true$none  WorkingFrames=Left$CS3$[0 0 0]$CS2$CS2$m$[0 0 0]$Euler X-Y-Z$deg$WORLD$true$none#Right$CS1$[0 0 0]$ADJOINING$ADJOINING$m$[0 0 0]$Euler X-Y-Z$deg$WORLD$true$none#Left$CS2$[-D12_S 0 0]$CS1$CS1$m$[0 0 0]$Euler X-Y-Z$deg$WORLD$true$none  CGPos=[D1G_S 0 0]  CGRot=[0 0 0]  CS0Pos=[]  CS0Rot=[]  CS1Pos=[0 0 0]  CS1Rot=[0 0 0]  CS2Pos=[-D12_S 0 0]  CS2Rot=[0 0 0]  CS3Pos=[0 0 0]  CS3Rot=[0 0 0]  CS4Pos=[]  CS4Rot=[]  CS5Pos=[]  CS5Rot=[]  CS6Pos=[]  CS6Rot=[]  CS7Pos=[]  CS7Rot=[]  CS8Pos=[]  CS8Rot=[]  CS9Pos=[]  CS9Rot=[]  CS10Pos=[]  CS10Rot=[]  CS11Pos=[]  CS11Rot=[]  CS12Pos=[]  CS12Rot=[]  CS13Pos=[]  CS13Rot=[]  CS14Pos=[]  CS14Rot=[]  CS15Pos=[]  CS15Rot=[]  CS16Pos=[]  CS16Rot=[]  CS17Pos=[]  CS17Rot=[]  CS18Pos=[]  CS18Rot=[]  CS19Pos=[]  CS19Rot=[]  CS20Pos=[]  CS20Rot=[]
      settings: SourceProductName=Simscape Multibody  SourceProductBaseCode=MS
  Right Thigh Sensor Sheet : Subsystem
  Right Thigh High : mblibv1/Bodies/Body  LConnTagsString=CS2  RConnTagsString=CS1  UpdateFromCAD=off  DialogClass=MechanicalBodyBlock  Mass=m_T*(1-ThPos)  MassUnits=kg  InertiaUnits=kg*m^2  Inertia=[Inx_T*(1-ThPos) 0 0; 0 Iny_T*(1-ThPos)^3 0; 0 0 In_T*(1-ThPos)^3]  Shape=Cylinder  ShapeDims=[1 1]  ShapeUnits=m  ShapeUse=false  Density=1  DensityUnits=kg/m^3  DensityUse=false  GraphicsMode=MACHINE_DEFAULT  BodyColorSelMode=MACHINE_DEFAULT  BodyColor=[1 0 0]  AttachedToCS=CG  CG=Left$CG$[-D1G_T*(1-ThPos) 0 0]$CS2$CS2$m$[0 0 0]$Euler X-Y-Z$deg$WORLD$false$none  WorkingFrames=Right$CS1$[0 0 0]$Adjoining$Adjoining$m$[0 0 0]$Euler X-Y-Z$deg$WORLD$true$none#Left$CS2$[D12_T*(1-ThPos) 0 0]$CS1$CS1$m$[0 0 0]$Euler X-Y-Z$deg$WORLD$true$none  CGPos=[-D1G_T*(1-ThPos) 0 0]  CGRot=[0 0 0]  CS0Pos=[]  CS0Rot=[]  CS1Pos=[0 0 0]  CS1Rot=[0 0 0]  CS2Pos=[D12_T*(1-ThPos) 0 0]  CS2Rot=[0 0 0]  CS3Pos=[]  CS3Rot=[]  CS4Pos=[]  CS4Rot=[]  CS5Pos=[]  CS5Rot=[]  CS6Pos=[]  CS6Rot=[]  CS7Pos=[]  CS7Rot=[]  CS8Pos=[]  CS8Rot=[]  CS9Pos=[]  CS9Rot=[]  CS10Pos=[]  CS10Rot=[]  CS11Pos=[]  CS11Rot=[]  CS12Pos=[]  CS12Rot=[]  CS13Pos=[]  CS13Rot=[]  CS14Pos=[]  CS14Rot=[]  CS15Pos=[]  CS15Rot=[]  CS16Pos=[]  CS16Rot=[]  CS17Pos=[]  CS17Rot=[]  CS18Pos=[]  CS18Rot=[]  CS19Pos=[]  CS19Rot=[]  CS20Pos=[]  CS20Rot=[]
      settings: SourceProductName=Simscape Multibody  SourceProductBaseCode=MS
  Right Thigh Low : mblibv1/Bodies/Body  LConnTagsString=CG|CS3|CS2  RConnTagsString=CS1  UpdateFromCAD=off  DialogClass=MechanicalBodyBlock  Mass=m_T*ThPos  MassUnits=kg  InertiaUnits=kg*m^2  Inertia=[Inx_T*ThPos 0 0; 0 Iny_T*(ThPos)^3 0; 0 0 In_T*(ThPos)^3]  Shape=Cylinder  ShapeDims=[1 1]  ShapeUnits=m  ShapeUse=false  Density=1  DensityUnits=kg/m^3  DensityUse=false  GraphicsMode=MACHINE_DEFAULT  BodyColorSelMode=MACHINE_DEFAULT  BodyColor=[1 0 0]  AttachedToCS=CG  CG=Left$CG$[-D1G_T*ThPos 0 0]$CS2$CS2$m$[0 0 0]$Euler X-Y-Z$deg$WORLD$true$none  WorkingFrames=Right$CS1$[0 0 0]$ADJOINING$ADJOINING$m$[0 0 0]$Euler X-Y-Z$deg$WORLD$true$none#Left$CS3$[0 0 0]$CS2$CS2$m$[0 0 0]$Euler X-Y-Z$deg$WORLD$true$none#Left$CS2$[D12_T*ThPos 0 0]$CS1$CS1$m$[0 0 0]$Euler X-Y-Z$deg$WORLD$true$none  CGPos=[-D1G_T*ThPos 0 0]  CGRot=[0 0 0]  CS0Pos=[]  CS0Rot=[]  CS1Pos=[0 0 0]  CS1Rot=[0 0 0]  CS2Pos=[D12_T*ThPos 0 0]  CS2Rot=[0 0 0]  CS3Pos=[0 0 0]  CS3Rot=[0 0 0]  CS4Pos=[]  CS4Rot=[]  CS5Pos=[]  CS5Rot=[]  CS6Pos=[]  CS6Rot=[]  CS7Pos=[]  CS7Rot=[]  CS8Pos=[]  CS8Rot=[]  CS9Pos=[]  CS9Rot=[]  CS10Pos=[]  CS10Rot=[]  CS11Pos=[]  CS11Rot=[]  CS12Pos=[]  CS12Rot=[]  CS13Pos=[]  CS13Rot=[]  CS14Pos=[]  CS14Rot=[]  CS15Pos=[]  CS15Rot=[]  CS16Pos=[]  CS16Rot=[]  CS17Pos=[]  CS17Rot=[]  CS18Pos=[]  CS18Rot=[]  CS19Pos=[]  CS19Rot=[]  CS20Pos=[]  CS20Rot=[]
      settings: SourceProductName=Simscape Multibody  SourceProductBaseCode=MS
  Scope : Scope
  Selector{,1..2,5..6} (5 alike) : Selector  InputPortWidth=3  IndexOptions=Index vector (dialog)  Indices=[1 2]  OutputSizes=1
  Selector{7,10,15..16} (4 alike) : Selector  InputPortWidth=3  IndexOptions=Index vector (dialog)  Indices=1  OutputSizes=1
  Selector{3..4,8..9,11..14} (8 alike) : Selector  InputPortWidth=3  IndexOptions=Index vector (dialog)  Indices=[1 3]  OutputSizes=1
  State sensor : Subsystem
  Terminator{,1..7} (8 alike) : Terminator
  To Workspace : ToWorkspace  VariableName=jointData  SaveFormat=Structure With Time  SampleTime=dt
  To Workspace1 : ToWorkspace  VariableName=RSwing  SaveFormat=Structure With Time  SampleTime=dt
  To Workspace2 : ToWorkspace  VariableName=stateData  SaveFormat=Structure With Time  SampleTime=dt
  Unit Delay4 : UnitDelay  SampleTime=-1  HasFrameUpgradeWarning=on
  body pitch/roll/yaw in body frame --- x-axis: forward y-axis: leftward z-axis: parallel to gravity : Subsystem
  "lateral d, v in body frame (left)" : Subsystem
  "lateral d, v in body frame (right)" : Subsystem
  map (-pi,pi] to [0,2pi){,3..7} (6 alike) : Fcn  Expr=u*(u>=0) + (2*pi+u)*(u<0)
  "sagittal d, v in body frame (left)" : Subsystem
  "sagittal d, v in body frame (right)" : Subsystem
  tag scope: LKneeState=global, LLBallCnt=global, LLHeelCnt=global, LLLoad=global, LMBallCnt=global, LMHeelCnt=global, Lphi12dphi12=global, Lphi23dphi23=global, Lphi34dphi34=global, Lphi34dphi34R=global, RKneeState=global, RLBallCnt=global, RLHeelCnt=global, RLLoad=global, RMBallCnt=global, RMHeelCnt=global, RSwing=global, Rphi12dphi12=global, Rphi23dphi23=global, Rphi34dphi34=global, Rphi34dphi34R=global, dtheta=global, dthetaR=global, dxyzHAT=global, dxyzLHip=global, dxyzRHip=global, front_dv_L=global, front_dv_R=global, side_dv_L=global, side_dv_R=global, theta=global, thetaR=global, thetaY=global, xyzHAT=global, xyzLAnkle=global, xyzLHip=global, xyzLKnee=global, xyzLLBall=global, xyzLLHeel=global, xyzLMBall=global, xyzLMHeel=global, xyzRAnkle=global, xyzRHip=global, xyzRKnee=global, xyzRLBall=global, xyzRLHeel=global, xyzRMBall=global, xyzRMHeel=global
  wires:
  Right Heel Sensor5/1 -> [xyzHAT]
  Right Heel Sensor5/2 -> [dxyzHAT]
  [LM12] -> Left Ankle Actuator/1
  [LM23] -> Left Knee Actuator/1
  Right Heel Sensor9/1 -> [xyzLHip]
  Right Heel Sensor9/2 -> [dxyzLHip]
  Right Heel Sensor8/2 -> [dxyzRHip]
  Right Heel Sensor8/1 -> [xyzRHip]
  LLHeel Cnt/1(RBallCnt) -> L Heel Skin Load Sensor/1
  L Heel Skin Load Sensor/1 -> [LLHeelCnt]
  L Ball Skin Load Sensor/1 -> [LLBallCnt]
  LLBall Cnt/1(RBallCnt) -> L Ball Skin Load Sensor/1
  Left Thigh Sensor Sheet/1(dx) -> L Thigh Displacement  Sensor/1
  L Thigh Displacement  Sensor/1 -> Left Leg Load/1(dxThigh [m])
  map (-pi,pi] to [0,2pi)6/1 -> Mux4/1
  LeftKnee Sensor/2 -> Mux4/2
  LeftKnee Sensor/1 -> map (-pi,pi] to [0,2pi)6/1
  Mux4/1 -> [Lphi23dphi23], L Knee Joint Sensor/1
  map (-pi,pi] to [0,2pi)3/1 -> Mux6/1
  Left Ankle Sensor/2 -> Mux6/2
  Left Ankle Sensor/1 -> map (-pi,pi] to [0,2pi)3/1
  Mux6/1 -> [Lphi12dphi12]
  L Knee Joint Sensor/1 -> [LKneeState]
  Right Heel Sensor7/1 -> [xyzLAnkle]
  [RM12] -> Right Ankle Actuator/1
  [RM23] -> Right Knee Actuator/1
  Right Thigh Sensor Sheet/1(dx) -> R Thigh Displacement  Sensor/1
  R Thigh Displacement  Sensor/1 -> Right Leg Load/1(dxThigh [m])
  map (-pi,pi] to [0,2pi)4/1 -> Mux5/1
  Right Knee Sensor/2 -> Mux5/2
  Mux5/1 -> [Rphi23dphi23], R Knee Joint Sensor/1
  Right Knee Sensor/1 -> map (-pi,pi] to [0,2pi)4/1
  map (-pi,pi] to [0,2pi)7/1 -> Mux7/1
  Right Ankle Sensor/2 -> Mux7/2
  Right Ankle Sensor/1 -> map (-pi,pi] to [0,2pi)7/1
  Mux7/1 -> [Rphi12dphi12]
  R Knee Joint Sensor/1 -> [RKneeState]
  Right Heel Sensor14/1 -> [xyzRKnee]
  Right Heel Sensor15/1 -> [xyzRAnkle]
  [LM34] -> Left Hip Actuator/1
  map (-pi,pi] to [0,2pi)/1 -> Mux2/1
  Left Hip Sensor/2 -> Mux2/2
  Left Hip Sensor/1 -> map (-pi,pi] to [0,2pi)/1
  Mux2/1 -> [Lphi34dphi34]
  Left Hip Sensor (roll)/2 -> Mux14/2
  Left Hip Sensor (roll)/1 -> Mux14/1
  Mux14/1 -> [Lphi34dphi34R]
  [LM34R] -> Left Hip Actuator (roll)/1
  [RM34] -> Right Hip Actuator/1
  map (-pi,pi] to [0,2pi)5/1 -> Mux3/1
  Right Hip Sensor/2 -> Mux3/2
  Right Hip Sensor/1 -> map (-pi,pi] to [0,2pi)5/1
  Mux3/1 -> [Rphi34dphi34]
  Right Hip Sensor (roll)/2 -> Mux15/2
  Right Hip Sensor (roll)/1 -> Mux15/1
  Mux15/1 -> L GLU Golgi Tendon Organs3/1
  [RM34R] -> L GLU Golgi Tendon Organs1/1
  L GLU Golgi Tendon Organs3/1 -> [Rphi34dphi34R]
  L GLU Golgi Tendon Organs1/1 -> Right Hip Actuator (roll)/1
  Right Heel Sensor21/1 -> [xyzLLBall]
  Right Heel Sensor20/1 -> [xyzLMBall]
  Right Heel Sensor23/1 -> [xyzLLHeel]
  Right Heel Sensor22/1 -> [xyzLMHeel]
  Right Heel Sensor12/1 -> [xyzRLHeel]
  Right Heel Sensor10/1 -> [xyzRMHeel]
  Right Heel Sensor3/1 -> [xyzRLBall]
  Right Heel Sensor13/1 -> [xyzRMBall]
  LMHeel Cnt/1(RBallCnt) -> L Heel Skin Load Sensor1/1
  L Heel Skin Load Sensor1/1 -> [LMHeelCnt]
  L Ball Skin Load Sensor1/1 -> [LMBallCnt]
  LMBall Cnt/1(RBallCnt) -> L Ball Skin Load Sensor1/1
  RLHeel Cnt/1(RBallCnt) -> L Heel Skin Load Sensor2/1
  RMHeel Cnt/1(RBallCnt) -> L Heel Skin Load Sensor3/1
  RMBall Cnt/1(RBallCnt) -> L Ball Skin Load Sensor3/1
  RLBall Cnt/1(RBallCnt) -> L Ball Skin Load Sensor2/1
  L Heel Skin Load Sensor2/1 -> [RLHeelCnt], OR/2
  L Heel Skin Load Sensor3/1 -> OR/3, [RMHeelCnt]
  L Ball Skin Load Sensor3/1 -> OR/4, [RMBallCnt]
  L Ball Skin Load Sensor2/1 -> [RLBallCnt], OR/1
  Right Heel Sensor6/1 -> [xyzLKnee]
  Left Leg Load/1(LLoad [F]) -> [LLLoad]
  Right Leg Load/1(LLoad [F]) -> [RLLoad]
  [xyzLAnkle] -> Selector9/1
  [xyzRAnkle] -> Selector11/1
  [dxyzHAT] -> Selector4/1
  Selector11/1 -> "lateral d, v in body frame (left)"/2(d0)
  Selector3/1 -> "lateral d, v in body frame (left)"/3(dist), "lateral d, v in body frame (right)"/3(dist)
  Selector4/1 -> "lateral d, v in body frame (left)"/4(vel), "lateral d, v in body frame (right)"/4(vel)
  [thetaY] -> "lateral d, v in body frame (left)"/1(body yaw), "lateral d, v in body frame (right)"/1(body yaw)
  [xyzHAT] -> Selector3/1
  Selector9/1 -> "lateral d, v in body frame (right)"/2(d0)
  body pitch/roll/yaw in body frame --- x-axis: forward y-axis: leftward z-axis: parallel to gravity/1(th_pitch) -> [theta]
  body pitch/roll/yaw in body frame --- x-axis: forward y-axis: leftward z-axis: parallel to gravity/2(dth_pitch) -> [dtheta]
  [xyzLHip] -> body pitch/roll/yaw in body frame --- x-axis: forward y-axis: leftward z-axis: parallel to gravity/1(LHip)
  [dxyzLHip] -> body pitch/roll/yaw in body frame --- x-axis: forward y-axis: leftward z-axis: parallel to gravity/2(dLHip)
  [xyzRHip] -> body pitch/roll/yaw in body frame --- x-axis: forward y-axis: leftward z-axis: parallel to gravity/5(RHip)
  [dxyzRHip] -> body pitch/roll/yaw in body frame --- x-axis: forward y-axis: leftward z-axis: parallel to gravity/6(dRHip)
  [xyzHAT] -> body pitch/roll/yaw in body frame --- x-axis: forward y-axis: leftward z-axis: parallel to gravity/3(HAT)
  [dxyzHAT] -> body pitch/roll/yaw in body frame --- x-axis: forward y-axis: leftward z-axis: parallel to gravity/4(dHAT)
  body pitch/roll/yaw in body frame --- x-axis: forward y-axis: leftward z-axis: parallel to gravity/3(th_roll) -> [thetaR]
  body pitch/roll/yaw in body frame --- x-axis: forward y-axis: leftward z-axis: parallel to gravity/4(dth_roll) -> [dthetaR]
  body pitch/roll/yaw in body frame --- x-axis: forward y-axis: leftward z-axis: parallel to gravity/5(yaw) -> [thetaY]
  "lateral d, v in body frame (left)"/1("d, v") -> L GLU Golgi Tendon Organs5/1
  [xyzLAnkle] -> Selector13/1
  [xyzRAnkle] -> Selector14/1
  [dxyzHAT] -> Selector12/1
  Selector14/1 -> "sagittal d, v in body frame (left)"/2(d0)
  Selector8/1 -> "sagittal d, v in body frame (left)"/3(dist), "sagittal d, v in body frame (right)"/3(dist)
  Selector12/1 -> "sagittal d, v in body frame (left)"/4(vel), "sagittal d, v in body frame (right)"/4(vel)
  [thetaY] -> "sagittal d, v in body frame (left)"/1(body yaw), "sagittal d, v in body frame (right)"/1(body yaw)
  [xyzHAT] -> Selector8/1
  Selector13/1 -> "sagittal d, v in body frame (right)"/2(d0)
  "sagittal d, v in body frame (left)"/1("d, v") -> [front_dv_L]
  "sagittal d, v in body frame (right)"/1("d, v") -> [front_dv_R]
  L GLU Golgi Tendon Organs5/1 -> [side_dv_L]
  "lateral d, v in body frame (right)"/1("d, v") -> [side_dv_R]
  LLHeel Cnt/2(GRF [N N N]) -> Terminator/1
  LMHeel Cnt/2(GRF [N N N]) -> Terminator1/1
  LMBall Cnt/2(GRF [N N N]) -> Terminator2/1
  LLBall Cnt/2(GRF [N N N]) -> Terminator3/1
  RLHeel Cnt/2(GRF [N N N]) -> Terminator4/1
  RMHeel Cnt/2(GRF [N N N]) -> Terminator5/1
  RMBall Cnt/2(GRF [N N N]) -> Terminator6/1
  RLBall Cnt/2(GRF [N N N]) -> Terminator7/1
  [xyzHAT] -> Selector/1
  [xyzRHip] -> Selector6/1
  [xyzRAnkle] -> Selector5/1
  [xyzLHip] -> Selector2/1
  [xyzLAnkle] -> Selector1/1
  Selector6/1 -> Mux/5
  Selector5/1 -> Mux/4
  Selector2/1 -> Mux/3
  Selector1/1 -> Mux/2
  Selector/1 -> Mux/1
  Mux/1 -> To Workspace/1
  OR/1 -> NOT/1
  NOT/1 -> Scope/1, [RSwing], To Workspace1/1
  [xyzLHip] -> Selector7/1
  Selector7/1 -> State sensor/1(In2)
  Selector10/1 -> State sensor/2(In3)
  [xyzRHip] -> Selector10/1
  [xyzRAnkle] -> Selector16/1
  [xyzLAnkle] -> Selector15/1
  Selector15/1 -> State sensor/3(In4)
  Selector16/1 -> State sensor/4(In5)
  Unit Delay4/1 -> Mux1/3
  Mux1/1 -> Controller/1
  Demux/2 -> Unit Delay4/1
  Demux/1 -> "Convert to torque "/1(In1)
  State sensor/1(x) -> To Workspace2/1, Mux1/1
  Controller/1 -> Demux/1
  [RSwing] -> Cast To Double/1
  Cast To Double/1 -> State sensor/5(In6)
  Clock/1 -> Mux1/2
  connections:
  HAT/RConn1 -- Left Hip Joint1/RConn1
  Left Foot/RConn3 -- Left Ankle Joint/LConn1
  Left Ankle Joint/LConn2 -- Left Ankle Actuator/RConn1
  Left Ankle Sensor/LConn1 -- Left Ankle Joint/LConn3
  Left Ankle Joint/RConn1 -- Left Shank/LConn2
  Left Ankle Joint/RConn2 -- Left Ankle IC/RConn1
  Left Hip Joint1/LConn1 -- Left Thigh High/LConn1
  Left Shank/RConn1 -- Left Knee Joint/LConn1
  Left Knee Joint/LConn2 -- Left Knee Actuator/RConn1
  LeftKnee Sensor/LConn1 -- Left Knee Joint/LConn3
  Left Knee Joint/RConn1 -- Left Thigh Low/RConn2
  Left Knee Joint/RConn2 -- Left Knee IC/RConn1
  Left Thigh Sensor Sheet/LConn1 -- Left Thigh Low/LConn1
  Left Thigh High/RConn1 -- Left Thigh Sensor Sheet/RConn1
  HAT/RConn2 -- Right Heel Sensor9/LConn1
  Right Heel Sensor5/LConn1 -- HAT/LConn1
  Ground/LConn1 -- Machine Environment/RConn1
  6 DOF/LConn1 -- Ground/RConn1
  HAT/RConn3 -- Right Heel Sensor8/LConn1
  Left Shank/LConn1 -- Right Heel Sensor7/LConn1
  Right Foot/RConn3 -- Right Ankle Joint/LConn1
  Right Ankle Actuator/RConn1 -- Right Ankle Joint/LConn2
  Right Ankle Joint/LConn3 -- Right Ankle Sensor/LConn1
  Right Ankle Joint/RConn1 -- Right Shank/LConn3
  Right Ankle Joint/RConn2 -- Right Ankle IC/RConn1
  Right Hip Joint1/LConn1 -- Right Thigh High/RConn1
  Right Shank/RConn1 -- Right Knee Joint/LConn1
  Right Knee Actuator/RConn1 -- Right Knee Joint/LConn2
  Right Knee Joint/LConn3 -- Right Knee Sensor/LConn1
  Right Knee Joint/RConn1 -- Right Thigh Low/LConn3
  Right Knee Joint/RConn2 -- Right Knee IC/RConn1
  HAT/RConn4 -- Right Hip Joint1/RConn1
  Right Heel Sensor15/LConn1 -- Right Shank/LConn2
  Right Thigh Sensor Sheet/LConn1 -- Right Thigh High/LConn1
  Right Thigh Sensor Sheet/RConn1 -- Right Thigh Low/RConn1
  Left Hip Joint1/LConn2 -- Left Hip Actuator/RConn1
  Left Hip Joint1/LConn3 -- Left Hip Sensor/LConn1
  Left Hip Joint1/RConn2 -- Left Hip IC/RConn1
  Left Hip Sensor (roll)/LConn1 -- Left Hip Joint1/RConn3
  Left Hip Actuator (roll)/RConn1 -- Left Hip Joint1/LConn4
  Right Hip Joint1/LConn2 -- Right Hip Actuator/RConn1
  Right Hip Joint1/LConn3 -- Right Hip Sensor/LConn1
  Right Hip IC/RConn1 -- Right Hip Joint1/RConn2
  Right Hip Actuator (roll)/RConn1 -- Right Hip Joint1/LConn4
  Right Hip Sensor (roll)/LConn1 -- Right Hip Joint1/RConn3
  6 DOF/LConn2 -- Left Ball IC/RConn1
  Left Foot/LConn1 -- Right Heel Sensor20/LConn1
  Left Foot/LConn2 -- Right Heel Sensor21/LConn1
  LLBall Cnt/LConn1 -- Left Foot/LConn4
  LMBall Cnt/LConn1 -- Left Foot/LConn5
  Left Foot/RConn1 -- Right Heel Sensor22/LConn1
  Left Foot/RConn2 -- Right Heel Sensor23/LConn1
  Left Foot/RConn4 -- LLHeel Cnt/LConn1
  LMHeel Cnt/LConn1 -- Left Foot/RConn5
  RMBall Cnt/LConn1 -- Right Foot/LConn5
  RLBall Cnt/LConn1 -- Right Foot/LConn4
  Right Foot/LConn1 -- Right Heel Sensor13/LConn1
  Right Foot/LConn2 -- Right Heel Sensor3/LConn1
  Right Heel Sensor10/LConn1 -- Right Foot/RConn1
  Right Foot/RConn2 -- Right Heel Sensor12/LConn1
  RMHeel Cnt/LConn1 -- Right Foot/RConn5
  RLHeel Cnt/LConn1 -- Right Foot/RConn4
  Left Foot/LConn3 -- 6 DOF/RConn1
  Left Thigh Low/RConn1 -- Right Heel Sensor6/LConn1
  Right Thigh Low/LConn2 -- Right Heel Sensor14/LConn1
  "Convert to torque "/RConn1 -- Right Shank/LConn1
